simulink model "w2_3"  (R2021a)
settings: Solver=VariableStepAuto  StartTime=0.0  StopTime=10.0  RelTol=1e-3
values from neighbouring files (symbols this model uses):
  b = 50.0    [w2_3.sldd]
  m = 1000.0    [w2_3.sldd]
settings Model: Creator=AVM  LastModifiedBy=AVM

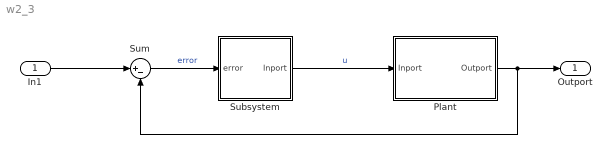
== system w2_3 ==
  In1 : Inport
  Plant : Subsystem
  Subsystem : Subsystem  TreatAsAtomicUnit=on
  Sum : Sum  Inputs=|+-
  Outport : Outport
  wires:
  Subsystem/1(Inport) -> Plant/1(Inport)  "u"
  Plant/1(Outport) -> Sum/2, Outport/1
  In1/1 -> Sum/1
  Sum/1 -> Subsystem/1(error)  "error"

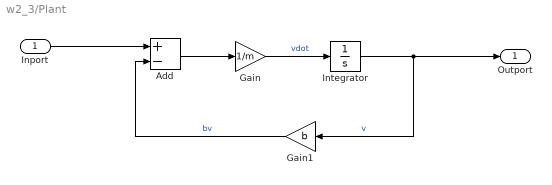
== system w2_3/Plant ==
  Inport : Inport
  Add : Sum  Inputs=+-
  Gain : Gain  Gain=1/m
  Gain1 : Gain  Gain=b
  Integrator : Integrator
  Outport : Outport
  wires:
  Inport/1 -> Add/1
  Integrator/1 -> Outport/1, Gain1/1  "v"
  Gain1/1 -> Add/2  "bv"
  Gain/1 -> Integrator/1  "vdot"
  Add/1 -> Gain/1

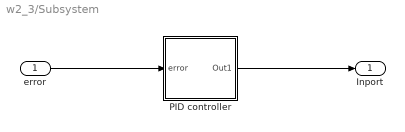
== system w2_3/Subsystem ==
  error : Inport
  PID controller : Subsystem  TreatAsAtomicUnit=on
  Inport : Outport
  wires:
  PID controller/1(Out1) -> Inport/1
  error/1 -> PID controller/1(error)

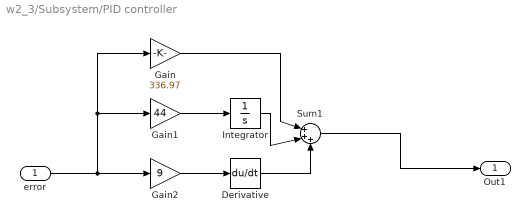
== system w2_3/Subsystem/PID controller ==
  error : Inport
  Derivative : Derivative
  Gain : Gain  Gain=336.97
  Gain1 : Gain  Gain=44
  Gain2 : Gain  Gain=9
  Integrator : Integrator
  Sum1 : Sum  Inputs=|+++
  Out1 : Outport
  wires:
  error/1 -> Gain2/1, Gain1/1, Gain/1
  Gain/1 -> Sum1/1
  Integrator/1 -> Sum1/2
  Gain1/1 -> Integrator/1
  Derivative/1 -> Sum1/3
  Sum1/1 -> Out1/1
  Gain2/1 -> Derivative/1
